simulink model "Q9_Simulation"  (R2022b)
settings: Solver=VariableStepAuto  StartTime=0.0  StopTime=25  RelTol=1e-3
undefined symbols (not defined in the file): A, B, C, K4, K5
settings Model: Creator=amirz  LastModifiedBy=amirz

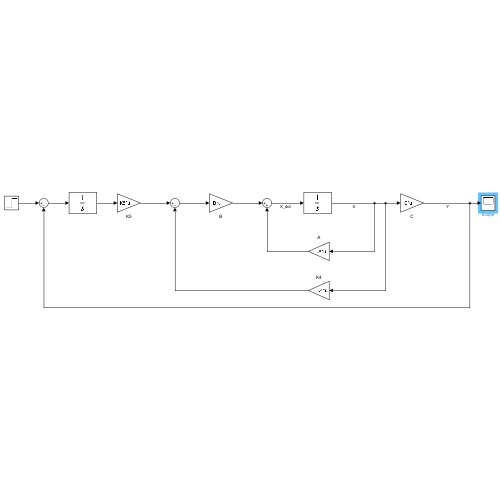
[thumbnail: Simulink's stored preview of the top-level diagram]
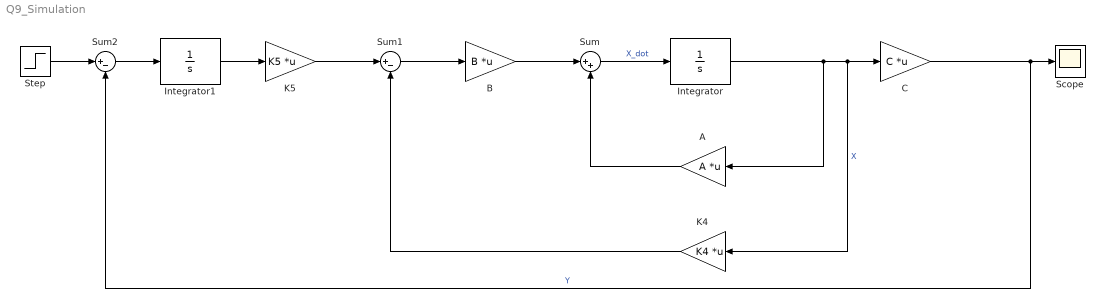
== system Q9_Simulation ==
  A : Gain  Gain=A  Multiplication=Matrix(K*u)
  B : Gain  Gain=B  Multiplication=Matrix(K*u)
  C : Gain  Gain=C  Multiplication=Matrix(K*u)
  Integrator : Integrator
  Integrator1 : Integrator
  K4 : Gain  Gain=K4  Multiplication=Matrix(K*u)
  K5 : Gain  Gain=K5  Multiplication=Matrix(K*u)
  Scope : Scope
  Step : Step  SampleTime=0
  Sum : Sum  Inputs=|++
  Sum1 : Sum  Inputs=|+-
  Sum2 : Sum  Inputs=|+-
  wires:
  C/1 -> Sum2/2, Scope/1  "Y"
  K5/1 -> Sum1/1
  K4/1 -> Sum1/2
  Integrator/1 -> A/1, K4/1, C/1  "X"
  Sum/1 -> Integrator/1  "X_dot"
  A/1 -> Sum/2
  Sum1/1 -> B/1
  B/1 -> Sum/1
  Integrator1/1 -> K5/1
  Sum2/1 -> Integrator1/1
  Step/1 -> Sum2/1
